simulink model "Lookuptabe1"  (R2025b)
settings: Solver=FixedStepDiscrete  StartTime=0.0  StopTime=1  FixedStep=0.0001  RelTol=1e-3
values from neighbouring files (symbols this model uses):
  A = 0.6*Xg.^2 - 0.4*Yg + 1.8*sin(2*Zg) + 0.15*Xg.*Yg.*sin(Zg) - 2.5    [test.m]    (also in test2.m = reshape(1:64, [4, 4, 4]))
  A1 = A(:)    [test.m]    (also in test2.m)
  X_dim = length(X_index)    [test.m]    (also in test2.m)
  X_index = linspace(-8.5, 12.3, 25)    [test.m]    (also in test2.m = X_index - 1.2)
  X_min = min(X_index)    [test.m]    (also in test2.m)
  X_step = X_index(2) - X_index(1)    [test.m]    (also in test2.m)
  XY_dim = X_dim * Y_dim    [test.m]    (also in test2.m)
  Y_dim = length(Y_index)    [test.m]    (also in test2.m)
  Y_index = linspace(-45.7, 67.2, 25)    [test.m]    (also in test2.m = Y_index - 2)
  Y_min = min(Y_index)    [test.m]    (also in test2.m)
  Y_step = Y_index(2) - Y_index(1)    [test.m]    (also in test2.m)
  Z_dim = length(Z_index)    [test.m]    (also in test2.m)
  Z_index = linspace(-3.8, 4.1, 25)    [test.m]    (also in test2.m = Z_index - 1)
  Z_min = min(Z_index)    [test.m]    (also in test2.m)
  Z_step = Z_index(2) - Z_index(1)    [test.m]    (also in test2.m)
settings Model: Creator=LXL1231A  LastModifiedBy=LXL1231A
settings OptimizationCC: DefaultParameterBehavior=Inlined  EnhancedBackFolding=on  PassReuseOutputArgsAs=Individual arguments  ZeroExternalMemoryAtStartup=off  ZeroInternalMemoryAtStartup=off  OptimizeBlockOrder=speed  DifferentSizesBufferReuse=on  OptimizationCustomize=off  EfficientTunableParamExpr=on
settings DebuggingCC: ParameterTunabilityLossMsg=error
settings SFSimCC: MATLABDynamicMemAlloc=off
settings RTWCC: SystemTargetFile=ert.tlc  GenCodeOnly=on  TemplateMakefile=ert_default_tmf  Description=Embedded Coder
settings CodeAppCC: ForceParamTrailComments=on  IgnoreCustomStorageClasses=off  OperatorAnnotations=on  SimulinkDataObjDesc=on  SFDataObjDesc=on  InsertBlockDesc=on
settings ERTTargetCC: ERTCustomFileTemplate=example_file_process.tlc  TargetLangStandard=C99 (ISO)  GenerateSampleERTMain=on

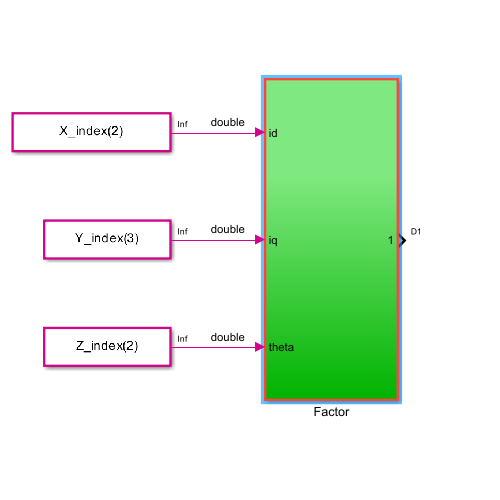
[thumbnail: Simulink's stored preview of the top-level diagram]
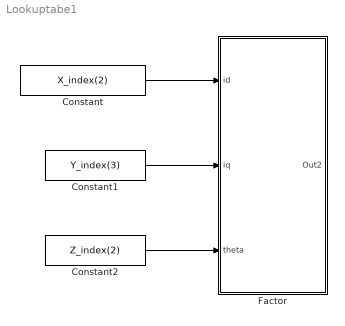
== system Lookuptabe1 ==
  Constant : Constant  Value=X_index(2)
  Constant1 : Constant  Value=Y_index(3)
  Constant2 : Constant  Value=Z_index(2)
  Factor : Subsystem
  wires:
  Constant/1 -> Factor/1(id)
  Constant1/1 -> Factor/2(iq)
  Constant2/1 -> Factor/3(theta)

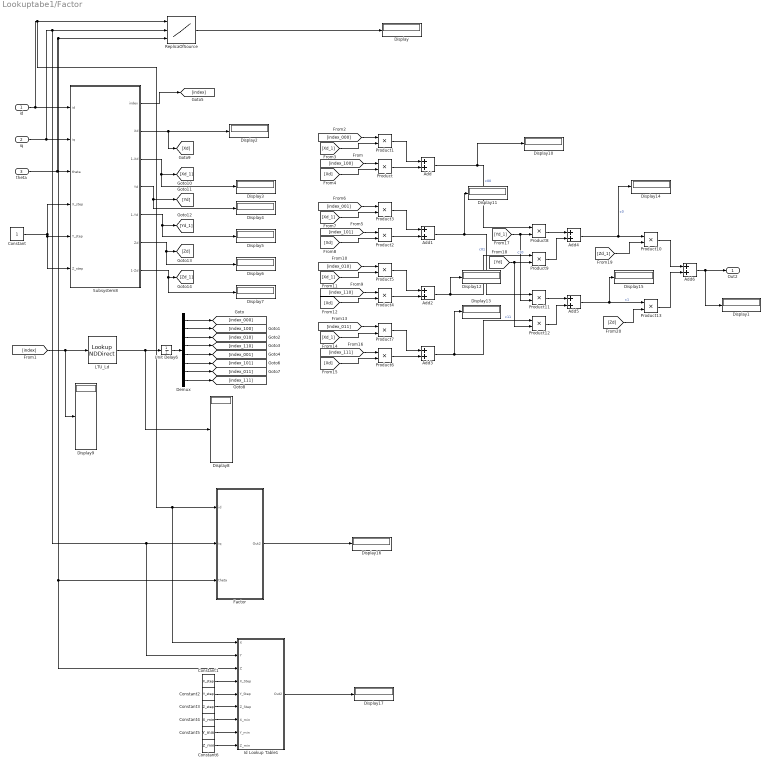
== system Lookuptabe1/Factor ==
  id : Inport
  iq : Inport  Port=2
  theta : Inport  Port=3
  Add{,1..6} (7 alike) : Sum
  Constant : Constant
  Constant1 : Constant  Value=X_step
  Constant2 : Constant  Value=Y_step
  Constant3 : Constant  Value=Z_step
  Constant4 : Constant  Value=X_min
  Constant5 : Constant  Value=Y_min
  Constant6 : Constant  Value=Z_min
  Demux : Demux  Outputs=8
  Display{,1..17} (18 alike) : Display
  Factor : Subsystem
  Id Lookup Table1 : Subsystem
  LTU_Ld : LookupNDDirect  NumberOfTableDimensions=1  Table=A1  TableDataTypeStr=fixdt(0,16,8)
  Product{,1..13} (14 alike) : Product
  ReplicaOfSource : Lookup_n-D  NumberOfTableDimensions=3  BreakpointsForDimension1=X_index  BreakpointsForDimension2=Y_index  BreakpointsForDimension3=Z_index  Table=A  InterpMethod=Linear Lagrange  InternalRulePriority=Speed  RndMeth=Simplest
      settings: InputPortMap=u0,u1,u2
  Subsystem8 : Subsystem
  Unit Delay6 : UnitDelay  SampleTime=-1  HasFrameUpgradeWarning=on
  Out2 : Outport
  wires:
  [index] -> Display9/1, LTU_Ld/1
  Subsystem8/1(index) -> [index]
  ReplicaOfSource/1 -> Display/1
  Constant/1 -> Subsystem8/6(Z_step), Subsystem8/5(Y_step), Subsystem8/4(X_step)
  Unit Delay6/1 -> Demux/1
  Demux/1 -> [index_000]
  [index_100] -> Product/1
  Product/1 -> Add/2
  Product1/1 -> Add/1
  [index_000] -> Product1/1
  Demux/2 -> [index_100]
  Demux/3 -> [index_010]
  Demux/4 -> [index_110]
  Demux/5 -> [index_001]
  Demux/6 -> [index_101]
  Demux/7 -> [index_011]
  Demux/8 -> [index_111]
  Subsystem8/2(Xd) -> [Xd], Display2/1
  Subsystem8/3(1-Xd) -> Display3/1, [Xd_1]
  Subsystem8/4(Yd) -> Display4/1, [Yd]
  Subsystem8/5(1-Yd) -> Display5/1, [Yd_1]
  Subsystem8/6(Zd) -> Display6/1, [Zd]
  Subsystem8/7(1-Zd) -> Display7/1, [Zd_1]
  [Xd_1] -> Product1/2
  [Xd] -> Product/2
  [index_101] -> Product2/1
  Product3/1 -> Add1/1
  Product2/1 -> Add1/2
  [index_001] -> Product3/1
  [Xd] -> Product2/2
  [Xd_1] -> Product3/2
  [index_010] -> Product5/1
  Product4/1 -> Add2/2
  Product5/1 -> Add2/1
  [Xd] -> Product4/2
  [index_110] -> Product4/1
  [Xd_1] -> Product5/2
  [Xd] -> Product6/2
  [index_111] -> Product6/1
  [index_011] -> Product7/1
  Product7/1 -> Add3/1
  Product6/1 -> Add3/2
  [Xd_1] -> Product7/2
  Add/1 -> Display10/1, Product8/1  "c00"
  [Yd_1] -> Product11/2, Product8/2
  Product8/1 -> Add4/1
  Product9/1 -> Add4/2
  Add2/1 -> Display12/1, Product9/1  "c10"
  [Yd] -> Product12/2, Product9/2
  Add4/1 -> Display14/1, Product10/1  "c0"
  [Zd_1] -> Product10/2
  Add1/1 -> Display11/1, Product11/1  "c01"
  Product11/1 -> Add5/1
  Add3/1 -> Display13/1, Product12/1  "c11"
  Product12/1 -> Add5/2
  Add5/1 -> Display15/1, Product13/1  "c1"
  [Zd] -> Product13/2
  Product10/1 -> Add6/1
  Product13/1 -> Add6/2
  Add6/1 -> Display1/1, Out2/1
  LTU_Ld/1 -> Display8/1, Unit Delay6/1
  Factor/1(Out2) -> Display16/1
  Constant1/1 -> Id Lookup Table1/4(X_Step)
  Id Lookup Table1/1(Out2) -> Display17/1
  Constant2/1 -> Id Lookup Table1/5(Y_Step)
  Constant3/1 -> Id Lookup Table1/6(Z_Step)
  Constant4/1 -> Id Lookup Table1/7(X_min)
  Constant5/1 -> Id Lookup Table1/8(Y_min)
  Constant6/1 -> Id Lookup Table1/9(Z_min)
  id/1 -> ReplicaOfSource/1, Id Lookup Table1/1(X), Factor/1(id), Subsystem8/1(id)
  iq/1 -> ReplicaOfSource/2, Id Lookup Table1/2(Y), Factor/2(iq), Subsystem8/2(iq)
  theta/1 -> ReplicaOfSource/3, Id Lookup Table1/3(Z), Factor/3(theta), Subsystem8/3(theta)

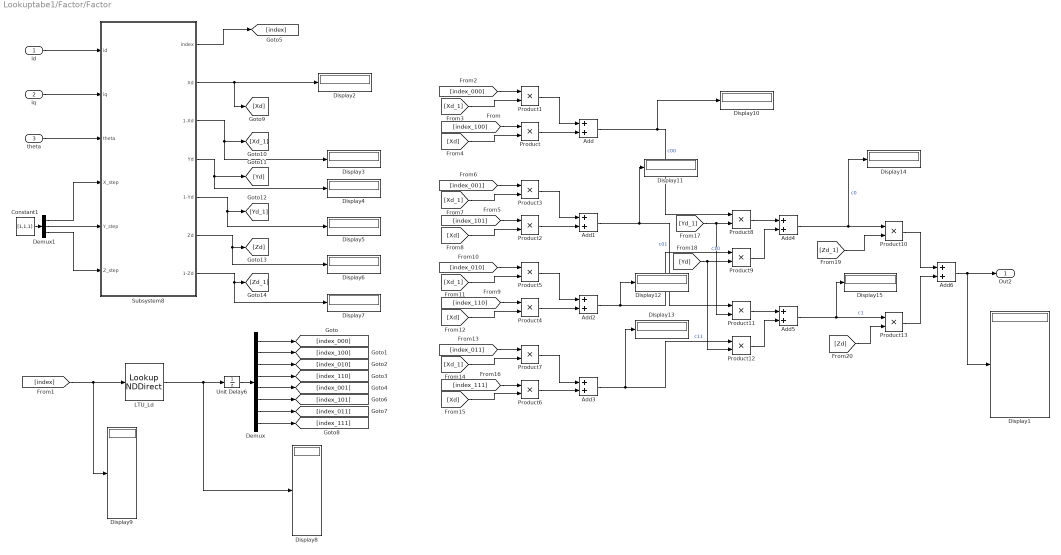
== system Lookuptabe1/Factor/Factor ==
  id : Inport
  iq : Inport  Port=2
  theta : Inport  Port=3
  Add{,1..6} (7 alike) : Sum
  Constant1 : Constant  Value=[1,1,1]
  Demux : Demux  Outputs=8
  Demux1 : Demux  Outputs=3
  Display{1..15} (15 alike) : Display
  LTU_Ld : LookupNDDirect  NumberOfTableDimensions=1  Table=A1  TableDataTypeStr=single
  Product{,1..13} (14 alike) : Product
  Subsystem8 : Subsystem
  Unit Delay6 : UnitDelay  SampleTime=-1  HasFrameUpgradeWarning=on
  Out2 : Outport
  wires:
  LTU_Ld/1 -> Unit Delay6/1, Display8/1
  Add6/1 -> Out2/1, Display1/1
  Product13/1 -> Add6/2
  Product10/1 -> Add6/1
  [Zd] -> Product13/2
  Add5/1 -> Product13/1, Display15/1  "c1"
  Product12/1 -> Add5/2
  Add3/1 -> Product12/1, Display13/1  "c11"
  Product11/1 -> Add5/1
  Add1/1 -> Product11/1, Display11/1  "c01"
  [Zd_1] -> Product10/2
  Add4/1 -> Product10/1, Display14/1  "c0"
  [Yd] -> Product9/2, Product12/2
  Add2/1 -> Product9/1, Display12/1  "c10"
  Product9/1 -> Add4/2
  Product8/1 -> Add4/1
  [Yd_1] -> Product8/2, Product11/2
  Add/1 -> Product8/1, Display10/1  "c00"
  [Xd_1] -> Product7/2
  Product6/1 -> Add3/2
  Product7/1 -> Add3/1
  [index_011] -> Product7/1
  [index_111] -> Product6/1
  [Xd] -> Product6/2
  [Xd_1] -> Product5/2
  [index_110] -> Product4/1
  [Xd] -> Product4/2
  Product5/1 -> Add2/1
  Product4/1 -> Add2/2
  [index_010] -> Product5/1
  [Xd_1] -> Product3/2
  [Xd] -> Product2/2
  [index_001] -> Product3/1
  Product2/1 -> Add1/2
  Product3/1 -> Add1/1
  [index_101] -> Product2/1
  [Xd] -> Product/2
  [Xd_1] -> Product1/2
  Subsystem8/7(1-Zd) -> [Zd_1], Display7/1
  Subsystem8/6(Zd) -> [Zd], Display6/1
  Subsystem8/5(1-Yd) -> [Yd_1], Display5/1
  Subsystem8/4(Yd) -> [Yd], Display4/1
  Subsystem8/3(1-Xd) -> [Xd_1], Display3/1
  Subsystem8/2(Xd) -> Display2/1, [Xd]
  Demux/8 -> [index_111]
  Demux/7 -> [index_011]
  Demux/6 -> [index_101]
  Demux/5 -> [index_001]
  Demux/4 -> [index_110]
  Demux/3 -> [index_010]
  Demux/2 -> [index_100]
  [index_000] -> Product1/1
  Product1/1 -> Add/1
  Product/1 -> Add/2
  [index_100] -> Product/1
  Demux/1 -> [index_000]
  Unit Delay6/1 -> Demux/1
  Subsystem8/1(index) -> [index]
  theta/1 -> Subsystem8/3(theta)
  iq/1 -> Subsystem8/2(iq)
  id/1 -> Subsystem8/1(id)
  [index] -> LTU_Ld/1, Display9/1
  Constant1/1 -> Demux1/1
  Demux1/1 -> Subsystem8/4(X_step)
  Demux1/2 -> Subsystem8/5(Y_step)
  Demux1/3 -> Subsystem8/6(Z_step)

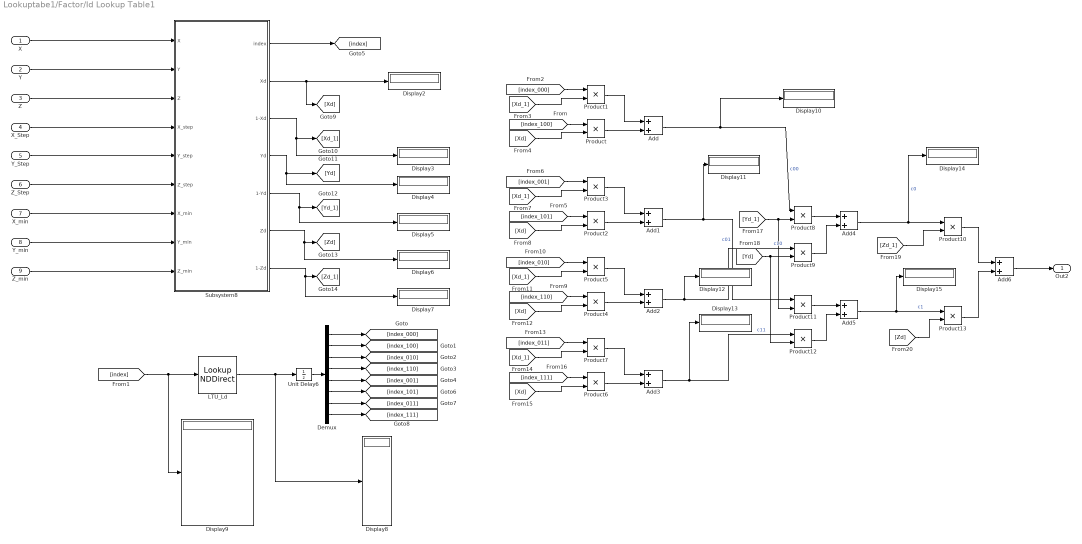
== system Lookuptabe1/Factor/Id Lookup Table1 ==
  X : Inport
  Y : Inport  Port=2
  Z : Inport  Port=3
  X_Step : Inport  Port=4
  Y_Step : Inport  Port=5
  Z_Step : Inport  Port=6
  X_min : Inport  Port=7
  Y_min : Inport  Port=8
  Z_min : Inport  Port=9
  Add{,1..6} (7 alike) : Sum
  Demux : Demux  Outputs=8
  Display{2..15} (14 alike) : Display
  LTU_Ld : LookupNDDirect  NumberOfTableDimensions=1  Table=A1  TableDataTypeStr=single
  Product{,1..13} (14 alike) : Product
  Subsystem8 : Subsystem
  Unit Delay6 : UnitDelay  SampleTime=-1  HasFrameUpgradeWarning=on
  Out2 : Outport
  wires:
  [index] -> Display9/1, LTU_Ld/1
  X/1 -> Subsystem8/1(X)
  Y/1 -> Subsystem8/2(Y)
  Z/1 -> Subsystem8/3(Z)
  Subsystem8/1(index) -> [index]
  Unit Delay6/1 -> Demux/1
  Demux/1 -> [index_000]
  [index_100] -> Product/1
  Product/1 -> Add/2
  Product1/1 -> Add/1
  [index_000] -> Product1/1
  Demux/2 -> [index_100]
  Demux/3 -> [index_010]
  Demux/4 -> [index_110]
  Demux/5 -> [index_001]
  Demux/6 -> [index_101]
  Demux/7 -> [index_011]
  Demux/8 -> [index_111]
  Subsystem8/2(Xd) -> [Xd], Display2/1
  Subsystem8/3(1-Xd) -> Display3/1, [Xd_1]
  Subsystem8/4(Yd) -> Display4/1, [Yd]
  Subsystem8/5(1-Yd) -> Display5/1, [Yd_1]
  Subsystem8/6(Zd) -> Display6/1, [Zd]
  Subsystem8/7(1-Zd) -> Display7/1, [Zd_1]
  [Xd_1] -> Product1/2
  [Xd] -> Product/2
  [index_101] -> Product2/1
  Product3/1 -> Add1/1
  Product2/1 -> Add1/2
  [index_001] -> Product3/1
  [Xd] -> Product2/2
  [Xd_1] -> Product3/2
  [index_010] -> Product5/1
  Product4/1 -> Add2/2
  Product5/1 -> Add2/1
  [Xd] -> Product4/2
  [index_110] -> Product4/1
  [Xd_1] -> Product5/2
  [Xd] -> Product6/2
  [index_111] -> Product6/1
  [index_011] -> Product7/1
  Product7/1 -> Add3/1
  Product6/1 -> Add3/2
  [Xd_1] -> Product7/2
  Add/1 -> Display10/1, Product8/1  "c00"
  [Yd_1] -> Product11/2, Product8/2
  Product8/1 -> Add4/1
  Product9/1 -> Add4/2
  Add2/1 -> Display12/1, Product9/1  "c10"
  [Yd] -> Product12/2, Product9/2
  Add4/1 -> Display14/1, Product10/1  "c0"
  [Zd_1] -> Product10/2
  Add1/1 -> Display11/1, Product11/1  "c01"
  Product11/1 -> Add5/1
  Add3/1 -> Display13/1, Product12/1  "c11"
  Product12/1 -> Add5/2
  Add5/1 -> Display15/1, Product13/1  "c1"
  [Zd] -> Product13/2
  Product10/1 -> Add6/1
  Product13/1 -> Add6/2
  Add6/1 -> Out2/1
  LTU_Ld/1 -> Display8/1, Unit Delay6/1
  X_Step/1 -> Subsystem8/4(X_step)
  Y_Step/1 -> Subsystem8/5(Y_step)
  Z_Step/1 -> Subsystem8/6(Z_step)
  X_min/1 -> Subsystem8/7(X_min)
  Z_min/1 -> Subsystem8/9(Z_min)
  Y_min/1 -> Subsystem8/8(Y_min)

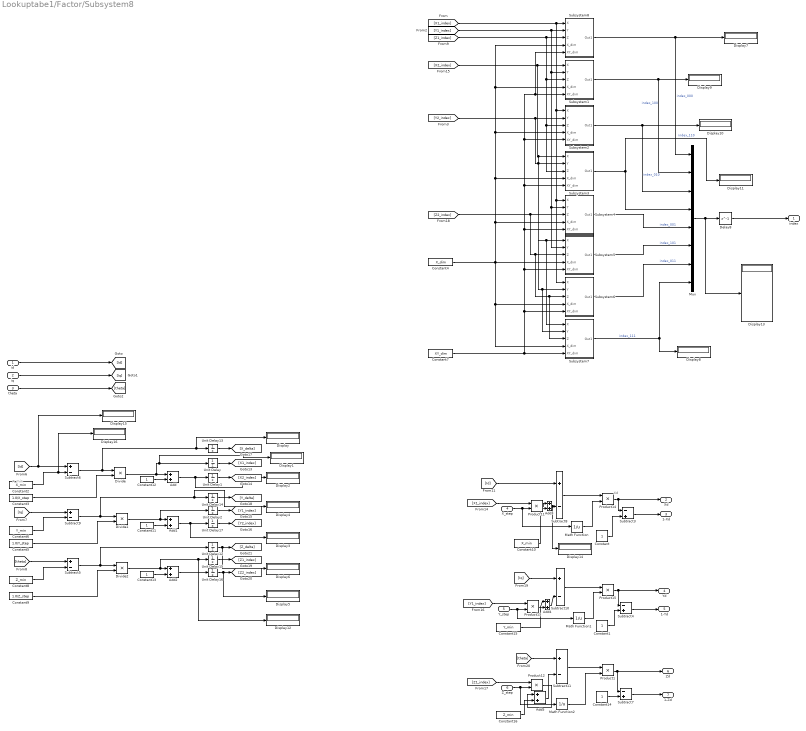
== system Lookuptabe1/Factor/Subsystem8 ==
  note: Xd
  note: X_min
  id : Inport
  iq : Inport  Port=2
  theta : Inport  Port=3
  X_step : Inport  Port=4
  Y_step : Inport  Port=5
  Z_step : Inport  Port=6
  Add : Sum  OutDataTypeStr=uint16
  Add1 : Sum  OutDataTypeStr=uint16
  Add2 : Sum  OutDataTypeStr=uint16
  Add3 : Sum
  Add4 : Sum
  Add5 : Sum
  Constant : Constant
  Constant1 : Constant
  Constant10 : Constant  Value=X_min  OutDataTypeStr=fixdt(1,LdLqTable_len,LdLqTable_fac)  SampleTime=-1
  Constant11 : Constant  OutDataTypeStr=uint16  SampleTime=-1
  Constant12 : Constant  OutDataTypeStr=uint16  SampleTime=-1
  Constant13 : Constant  OutDataTypeStr=uint16  SampleTime=-1
  Constant14 : Constant
  Constant15 : Constant  Value=Y_min  OutDataTypeStr=fixdt(1,LdLqTable_len,LdLqTable_fac)  SampleTime=-1
  Constant16 : Constant  Value=Z_min  OutDataTypeStr=fixdt(1,LdLqTable_len,LdLqTable_fac)  SampleTime=-1
  Constant2 : Constant  Value=X_min  OutDataTypeStr=fixdt(1,LdLqTable_len,LdLqTable_fac)  SampleTime=-1
  Constant3 : Constant  Value=1.0/X_step  OutDataTypeStr=fixdt(1,LdLqTable_len,LdLqTable_fac)  SampleTime=-1
  Constant4 : Constant  Value=X_dim  OutDataTypeStr=uint16  SampleTime=-1
  Constant5 : Constant  Value=1.0/Y_step  OutDataTypeStr=fixdt(1,LdLqTable_len,LdLqTable_fac)  SampleTime=-1
  Constant6 : Constant  Value=Y_min  OutDataTypeStr=fixdt(1,LdLqTable_len,LdLqTable_fac)  SampleTime=-1
  Constant7 : Constant  Value=XY_dim  OutDataTypeStr=uint16  SampleTime=-1
  Constant8 : Constant  Value=Z_min  OutDataTypeStr=fixdt(1,LdLqTable_len,LdLqTable_fac)  SampleTime=-1
  Constant9 : Constant  Value=1.0/Z_step  OutDataTypeStr=fixdt(1,LdLqTable_len,LdLqTable_fac)  SampleTime=-1
  Delay8 : Delay  DelayLength=1
  Display{,1..16} (17 alike) : Display
  Divide : Product  OutDataTypeStr=uint16
  Divide1 : Product  OutDataTypeStr=uint16
  Divide2 : Product  OutDataTypeStr=uint16
  Math Function : Math  Operator=reciprocal
  Math Function1 : Math  Operator=reciprocal
  Math Function2 : Math  Operator=reciprocal
  Mux : Mux  Inputs=8
  Product1 : Product
  Product11 : Product  OutDataTypeStr=fixdt(1,LdLqTable_len,LdLqTable_fac)
  Product12 : Product  OutDataTypeStr=fixdt(1,LdLqTable_len,LdLqTable_fac)
  Product13 : Product  OutDataTypeStr=fixdt(1,LdLqTable_len,LdLqTable_fac)
  Product14 : Product
  Product15 : Product
  Subsystem1 : Subsystem
  Subsystem2 : Subsystem
  Subsystem3 : Subsystem
  Subsystem4 : Subsystem
  Subsystem5 : Subsystem
  Subsystem6 : Subsystem
  Subsystem7 : Subsystem
  Subsystem8 : Subsystem
  Subtract10 : Sum  Inputs=+-  OutDataTypeStr=fixdt(1,LdLqTable_len,LdLqTable_fac)
  Subtract11 : Sum  Inputs=+-  OutDataTypeStr=fixdt(1,LdLqTable_len,LdLqTable_fac)
  Subtract3 : Sum  Inputs=-+
  Subtract4 : Sum  Inputs=-+
  Subtract5 : Sum  Inputs=+-  OutDataTypeStr=fixdt(1,Id_lim_len,Id_lim_fac)
  Subtract6 : Sum  Inputs=+-  OutDataTypeStr=fixdt(1,Id_lim_len,Id_lim_fac)
  Subtract7 : Sum  Inputs=-+
  Subtract8 : Sum  Inputs=+-  OutDataTypeStr=fixdt(1,LdLqTable_len,LdLqTable_fac)
  Subtract9 : Sum  Inputs=+-  OutDataTypeStr=fixdt(1,Id_lim_len,Id_lim_fac)
  Unit Delay{,1..2,12..17} (9 alike) : UnitDelay  SampleTime=-1  HasFrameUpgradeWarning=on
  index : Outport
  Xd : Outport  Port=2
  1-Xd : Outport  Port=3
  Yd : Outport  Port=4
  1-Yd : Outport  Port=5
  Zd : Outport  Port=6
  1-Zd : Outport  Port=7
  wires:
  Constant9/1 -> Divide2/2
  Subtract6/1 -> Display/1, Unit Delay13/1, Divide/1
  Mux/1 -> Display13/1, Delay8/1
  Unit Delay16/1 -> Display5/1, [Z2_index]
  [Z2_index] -> Subsystem4/3(Z), Subsystem5/3(Z), Subsystem7/3(Z), Subsystem6/3(Z)
  [X1_index] -> Subsystem8/1(X), Subsystem2/1(X), Subsystem6/1(X), Subsystem4/1(X)
  Divide/1 -> Unit Delay/1, Display1/1, Add/1
  Constant8/1 -> Subtract5/2
  Unit Delay2/1 -> [Y1_index]
  Unit Delay13/1 -> [X_delta]
  Constant4/1 -> Subsystem8/4(X_dim), Subsystem1/4(X_dim), Subsystem2/4(X_dim), Subsystem3/4(X_dim), Subsystem4/4(X_dim), Subsystem5/4(X_dim), Subsystem7/4(X_dim), Subsystem6/4(X_dim)
  Unit Delay12/1 -> Display6/1, [Z_delta]
  Constant7/1 -> Subsystem6/5(XY_dim), Subsystem5/5(XY_dim), Subsystem4/5(XY_dim), Subsystem3/5(XY_dim), Subsystem2/5(XY_dim), Subsystem1/5(XY_dim), Subsystem8/5(XY_dim), Subsystem7/5(XY_dim)
  Constant13/1 -> Add2/2
  Divide1/1 -> Unit Delay2/1, Add1/1
  Constant12/1 -> Add/2
  [Y2_index] -> Subsystem2/2(Y), Subsystem3/2(Y), Subsystem7/2(Y), Subsystem6/2(Y)
  Subtract9/1 -> Divide1/1, Display4/1, Unit Delay14/1
  Unit Delay/1 -> [X1_index]
  Constant11/1 -> Add1/2
  Unit Delay1/1 -> [X2_index]
  Unit Delay15/1 -> [Z1_index]
  Subsystem2/1(Out1) -> Display10/1, Mux/3  "index_010"
  Subsystem8/1(Out1) -> Display7/1, Mux/1  "index_000"
  Add1/1 -> Display3/1, Unit Delay17/1
  Constant2/1 -> Display16/1, Subtract6/2
  Subsystem1/1(Out1) -> Display9/1, Mux/2  "index_100"
  Unit Delay14/1 -> [Y_delta]
  Subsystem3/1(Out1) -> Mux/4, Display11/1  "index_110"
  [X2_index] -> Subsystem1/1(X), Subsystem3/1(X), Subsystem7/1(X), Subsystem5/1(X)
  Constant6/1 -> Subtract9/2
  Unit Delay17/1 -> [Y2_index]
  Constant3/1 -> Divide/2
  Subsystem7/1(Out1) -> Mux/8, Display8/1  "index_111"
  [Z1_index] -> Subsystem8/3(Z), Subsystem1/3(Z), Subsystem3/3(Z), Subsystem2/3(Z)
  Constant5/1 -> Divide1/2
  Add/1 -> Display2/1, Unit Delay1/1
  Delay8/1 -> index/1
  Subtract5/1 -> Divide2/1, Unit Delay12/1
  Add2/1 -> Unit Delay16/1
  Subsystem6/1(Out1) -> Mux/7  "index_011"
  Subsystem4/1(Out1) -> Mux/5  "index_001"
  [Y1_index] -> Subsystem8/2(Y), Subsystem1/2(Y), Subsystem5/2(Y), Subsystem4/2(Y)
  Divide2/1 -> Display12/1, Unit Delay15/1, Add2/1
  Subsystem5/1(Out1) -> Mux/6  "index_101"
  [Iq] -> Subtract9/1
  [theta] -> Subtract5/1
  id/1 -> [Id]
  iq/1 -> [Iq]
  theta/1 -> [theta]
  [Id] -> Subtract8/1
  Product11/1 -> Add3/1
  [theta] -> Subtract11/1
  [X1_index] -> Product11/1
  Y_step/1 -> Math Function1/1, Product13/2
  [Iq] -> Subtract10/1
  Z_step/1 -> Math Function2/1, Product12/2
  Product12/1 -> Add5/1
  X_step/1 -> Math Function/1, Product11/2
  [Y1_index] -> Product13/1
  [Z1_index] -> Product12/1
  Product13/1 -> Add4/1
  Subtract8/1 -> Product14/1
  Math Function/1 -> Product14/2
  Subtract10/1 -> Product15/1
  Math Function1/1 -> Product15/2
  Math Function2/1 -> Product1/2
  Subtract11/1 -> Product1/1
  Product14/1 -> Subtract3/1, Xd/1
  Product15/1 -> Subtract4/1, Yd/1
  Product1/1 -> Subtract7/1, Zd/1
  Subtract3/1 -> 1-Xd/1
  Constant/1 -> Subtract3/2
  Subtract4/1 -> 1-Yd/1
  Constant1/1 -> Subtract4/2
  Subtract7/1 -> 1-Zd/1
  Constant14/1 -> Subtract7/2
  Add3/1 -> Display14/1, Subtract8/2
  Constant10/1 -> Add3/2
  Add4/1 -> Subtract10/2
  Constant15/1 -> Add4/2
  Constant16/1 -> Add5/2
  Add5/1 -> Subtract11/2
  [Id] -> Display15/1, Subtract6/1

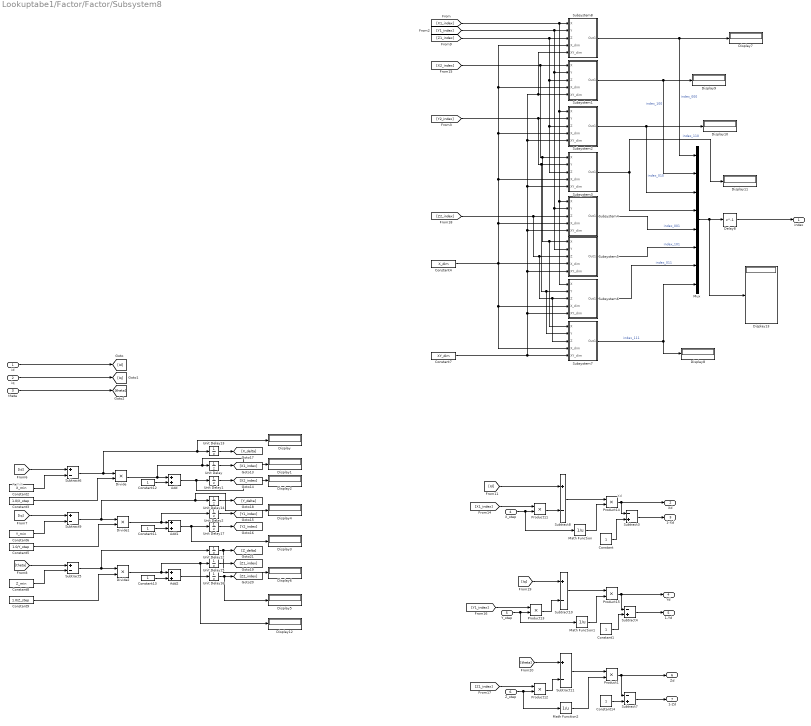
== system Lookuptabe1/Factor/Factor/Subsystem8 ==
  note: X_min
  note: Xd
  id : Inport
  iq : Inport  Port=2
  theta : Inport  Port=3
  X_step : Inport  Port=4
  Y_step : Inport  Port=5
  Z_step : Inport  Port=6
  Add : Sum
  Add1 : Sum  OutDataTypeStr=single
  Add2 : Sum  OutDataTypeStr=single  AccumDataTypeStr=single
  Constant : Constant
  Constant1 : Constant
  Constant11 : Constant  OutDataTypeStr=uint32  SampleTime=-1
  Constant12 : Constant  OutDataTypeStr=uint32  SampleTime=-1
  Constant13 : Constant  OutDataTypeStr=uint32  SampleTime=-1
  Constant14 : Constant
  Constant2 : Constant  Value=X_min  OutDataTypeStr=single  SampleTime=-1
  Constant3 : Constant  Value=1.0/X_step  OutDataTypeStr=single  SampleTime=-1
  Constant4 : Constant  Value=X_dim  OutDataTypeStr=single  SampleTime=-1
  Constant5 : Constant  Value=1.0/Y_step  OutDataTypeStr=single  SampleTime=-1
  Constant6 : Constant  Value=Y_min  OutDataTypeStr=single  SampleTime=-1
  Constant7 : Constant  Value=XY_dim  OutDataTypeStr=single  SampleTime=-1
  Constant8 : Constant  Value=Z_min  OutDataTypeStr=single  SampleTime=-1
  Constant9 : Constant  Value=1.0/Z_step  OutDataTypeStr=single  SampleTime=-1
  Delay8 : Delay  DelayLength=1
  Display{,1..13} (14 alike) : Display
  Divide : Product  OutDataTypeStr=uint16
  Divide1 : Product  OutDataTypeStr=uint16
  Divide2 : Product  OutDataTypeStr=uint16
  Math Function : Math  Operator=reciprocal
  Math Function1 : Math  Operator=reciprocal
  Math Function2 : Math  Operator=reciprocal
  Mux : Mux  Inputs=8
  Product1 : Product
  Product11 : Product  OutDataTypeStr=single
  Product12 : Product  OutDataTypeStr=single
  Product13 : Product  OutDataTypeStr=single
  Product14 : Product
  Product15 : Product
  Subsystem1 : Subsystem
  Subsystem2 : Subsystem
  Subsystem3 : Subsystem
  Subsystem4 : Subsystem
  Subsystem5 : Subsystem
  Subsystem6 : Subsystem
  Subsystem7 : Subsystem
  Subsystem8 : Subsystem
  Subtract{5..6,8..11} (6 alike) : Sum  Inputs=+-  OutDataTypeStr=single
  Subtract3 : Sum  Inputs=-+
  Subtract4 : Sum  Inputs=-+
  Subtract7 : Sum  Inputs=-+
  Unit Delay{,1..2,12..17} (9 alike) : UnitDelay  SampleTime=-1  HasFrameUpgradeWarning=on
  index : Outport
  Xd : Outport  Port=2
  1-Xd : Outport  Port=3
  Yd : Outport  Port=4
  1-Yd : Outport  Port=5
  Zd : Outport  Port=6
  1-Zd : Outport  Port=7
  wires:
  Constant14/1 -> Subtract7/2
  Subtract7/1 -> 1-Zd/1
  Constant1/1 -> Subtract4/2
  Subtract4/1 -> 1-Yd/1
  Constant/1 -> Subtract3/2
  Subtract3/1 -> 1-Xd/1
  Product1/1 -> Zd/1, Subtract7/1
  Product15/1 -> Yd/1, Subtract4/1
  Product14/1 -> Xd/1, Subtract3/1
  Subtract11/1 -> Product1/1
  Math Function2/1 -> Product1/2
  Math Function1/1 -> Product15/2
  Subtract10/1 -> Product15/1
  Math Function/1 -> Product14/2
  Subtract8/1 -> Product14/1
  Product13/1 -> Subtract10/2
  [Z1_index] -> Product12/1
  [Y1_index] -> Product13/1
  X_step/1 -> Product11/2, Math Function/1
  Product12/1 -> Subtract11/2
  Z_step/1 -> Product12/2, Math Function2/1
  [Iq] -> Subtract10/1
  Y_step/1 -> Product13/2, Math Function1/1
  [X1_index] -> Product11/1
  [theta] -> Subtract11/1
  Product11/1 -> Subtract8/2
  [Id] -> Subtract8/1
  theta/1 -> [theta]
  iq/1 -> [Iq]
  id/1 -> [Id]
  [theta] -> Subtract5/1
  [Iq] -> Subtract9/1
  [Id] -> Subtract6/1
  Subsystem5/1(Out1) -> Mux/6  "index_101"
  Divide2/1 -> Add2/1, Unit Delay15/1, Display12/1
  [Y1_index] -> Subsystem5/2(Y), Subsystem4/2(Y), Subsystem1/2(Y), Subsystem8/2(Y)
  Subsystem4/1(Out1) -> Mux/5  "index_001"
  Subsystem6/1(Out1) -> Mux/7  "index_011"
  Add2/1 -> Unit Delay16/1
  Subtract5/1 -> Unit Delay12/1, Divide2/1
  Delay8/1 -> index/1
  Add/1 -> Unit Delay1/1, Display2/1
  Constant5/1 -> Divide1/2
  [Z1_index] -> Subsystem3/3(Z), Subsystem2/3(Z), Subsystem1/3(Z), Subsystem8/3(Z)
  Subsystem7/1(Out1) -> Display8/1, Mux/8  "index_111"
  Constant3/1 -> Divide/2
  Unit Delay17/1 -> [Y2_index]
  Constant6/1 -> Subtract9/2
  [X2_index] -> Subsystem3/1(X), Subsystem7/1(X), Subsystem5/1(X), Subsystem1/1(X)
  Subsystem3/1(Out1) -> Display11/1, Mux/4  "index_110"
  Unit Delay14/1 -> [Y_delta]
  Subsystem1/1(Out1) -> Mux/2, Display9/1  "index_100"
  Constant2/1 -> Subtract6/2
  Add1/1 -> Unit Delay17/1, Display3/1
  Subsystem8/1(Out1) -> Mux/1, Display7/1  "index_000"
  Subsystem2/1(Out1) -> Mux/3, Display10/1  "index_010"
  Unit Delay15/1 -> [Z1_index]
  Unit Delay1/1 -> [X2_index]
  Constant11/1 -> Add1/2
  Unit Delay/1 -> [X1_index]
  Subtract9/1 -> Unit Delay14/1, Display4/1, Divide1/1
  [Y2_index] -> Subsystem2/2(Y), Subsystem3/2(Y), Subsystem7/2(Y), Subsystem6/2(Y)
  Constant12/1 -> Add/2
  Divide1/1 -> Add1/1, Unit Delay2/1
  Constant13/1 -> Add2/2
  Constant7/1 -> Subsystem7/5(XY_dim), Subsystem6/5(XY_dim), Subsystem5/5(XY_dim), Subsystem4/5(XY_dim), Subsystem3/5(XY_dim), Subsystem2/5(XY_dim), Subsystem8/5(XY_dim), Subsystem1/5(XY_dim)
  Unit Delay12/1 -> [Z_delta], Display6/1
  Constant4/1 -> Subsystem5/4(X_dim), Subsystem7/4(X_dim), Subsystem6/4(X_dim), Subsystem4/4(X_dim), Subsystem3/4(X_dim), Subsystem2/4(X_dim), Subsystem1/4(X_dim), Subsystem8/4(X_dim)
  Unit Delay13/1 -> [X_delta]
  Unit Delay2/1 -> [Y1_index]
  Constant8/1 -> Subtract5/2
  Divide/1 -> Add/1, Unit Delay/1, Display1/1
  [X1_index] -> Subsystem2/1(X), Subsystem6/1(X), Subsystem4/1(X), Subsystem8/1(X)
  [Z2_index] -> Subsystem4/3(Z), Subsystem5/3(Z), Subsystem7/3(Z), Subsystem6/3(Z)
  Unit Delay16/1 -> [Z2_index], Display5/1
  Mux/1 -> Delay8/1, Display13/1
  Subtract6/1 -> Divide/1, Unit Delay13/1, Display/1
  Constant9/1 -> Divide2/2

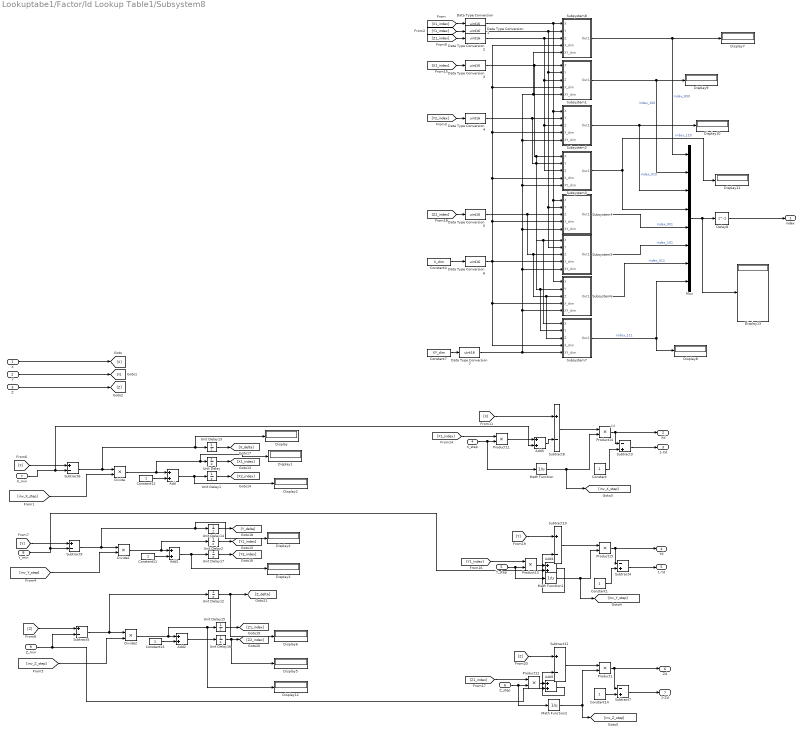
== system Lookuptabe1/Factor/Id Lookup Table1/Subsystem8 ==
  note: Xd
  X : Inport
  Y : Inport  Port=2
  Z : Inport  Port=3
  X_step : Inport  Port=4
  Y_step : Inport  Port=5
  Z_step : Inport  Port=6
  X_min : Inport  Port=7
  Y_min : Inport  Port=8
  Z_min : Inport  Port=9
  Add{,3..5} (4 alike) : Sum
  Add1 : Sum  OutDataTypeStr=single
  Add2 : Sum  OutDataTypeStr=single  AccumDataTypeStr=single
  Constant : Constant
  Constant1 : Constant
  Constant11 : Constant  OutDataTypeStr=uint32  SampleTime=-1
  Constant12 : Constant  OutDataTypeStr=uint32  SampleTime=-1
  Constant13 : Constant  OutDataTypeStr=uint32  SampleTime=-1
  Constant14 : Constant
  Constant4 : Constant  Value=X_dim  OutDataTypeStr=single  SampleTime=-1
  Constant7 : Constant  Value=XY_dim  OutDataTypeStr=single  SampleTime=-1
  Data Type Conversion{,1..7} (8 alike) : DataTypeConversion  OutDataTypeStr=uint16  SaturateOnIntegerOverflow=off  RndMeth=Floor
  Delay8 : Delay  DelayLength=1
  Display{,1..13} (14 alike) : Display
  Divide : Product  OutDataTypeStr=single
  Divide1 : Product  OutDataTypeStr=single
  Divide2 : Product  OutDataTypeStr=single
  Math Function : Math  Operator=reciprocal
  Math Function1 : Math  Operator=reciprocal
  Math Function2 : Math  Operator=reciprocal
  Mux : Mux  Inputs=8
  Product1 : Product
  Product11 : Product  OutDataTypeStr=single
  Product12 : Product  OutDataTypeStr=single
  Product13 : Product  OutDataTypeStr=single
  Product14 : Product
  Product15 : Product
  Subsystem1 : Subsystem
  Subsystem2 : Subsystem
  Subsystem3 : Subsystem
  Subsystem4 : Subsystem
  Subsystem5 : Subsystem
  Subsystem6 : Subsystem
  Subsystem7 : Subsystem
  Subsystem8 : Subsystem
  Subtract{5..6,8..11} (6 alike) : Sum  Inputs=+-  OutDataTypeStr=single
  Subtract3 : Sum  Inputs=-+
  Subtract4 : Sum  Inputs=-+
  Subtract7 : Sum  Inputs=-+
  Unit Delay{,1..2,12..17} (9 alike) : UnitDelay  SampleTime=-1  HasFrameUpgradeWarning=on
  index : Outport
  Xd : Outport  Port=2
  1-Xd : Outport  Port=3
  Yd : Outport  Port=4
  1-Yd : Outport  Port=5
  Zd : Outport  Port=6
  1-Zd : Outport  Port=7
  wires:
  [inv_Z_step] -> Divide2/2
  Subtract6/1 -> Display/1, Unit Delay13/1, Divide/1
  Mux/1 -> Display13/1, Delay8/1
  Unit Delay16/1 -> Display5/1, [Z2_index]
  [Z2_index] -> Data Type Conversion5/1
  [X1_index] -> Data Type Conversion/1
  Divide/1 -> Display1/1, Unit Delay/1, Add/1
  Unit Delay2/1 -> [Y1_index]
  Unit Delay13/1 -> [X_delta]
  Constant4/1 -> Data Type Conversion6/1
  Unit Delay12/1 -> Display6/1, [Z_delta]
  Constant7/1 -> Data Type Conversion7/1
  Constant13/1 -> Add2/2
  Divide1/1 -> Unit Delay2/1, Add1/1
  Constant12/1 -> Add/2
  [Y2_index] -> Data Type Conversion4/1
  Subtract9/1 -> Divide1/1, Display4/1, Unit Delay14/1
  Unit Delay/1 -> [X1_index]
  Constant11/1 -> Add1/2
  Unit Delay1/1 -> [X2_index]
  Unit Delay15/1 -> [Z1_index]
  Subsystem2/1(Out1) -> Display10/1, Mux/3  "index_010"
  Subsystem8/1(Out1) -> Display7/1, Mux/1  "index_000"
  Add1/1 -> Display3/1, Unit Delay17/1
  X_min/1 -> Add3/2, Subtract6/2
  Subsystem1/1(Out1) -> Display9/1, Mux/2  "index_100"
  Unit Delay14/1 -> [Y_delta]
  Subsystem3/1(Out1) -> Mux/4, Display11/1  "index_110"
  [X2_index] -> Data Type Conversion3/1
  Unit Delay17/1 -> [Y2_index]
  [inv_X_step] -> Divide/2
  Subsystem7/1(Out1) -> Mux/8, Display8/1  "index_111"
  [Z1_index] -> Data Type Conversion2/1
  [inv_Y_step] -> Divide1/2
  Add/1 -> Display2/1, Unit Delay1/1
  Delay8/1 -> index/1
  Subtract5/1 -> Divide2/1, Unit Delay12/1
  Add2/1 -> Unit Delay16/1
  Subsystem6/1(Out1) -> Mux/7  "index_011"
  Subsystem4/1(Out1) -> Mux/5  "index_001"
  [Y1_index] -> Data Type Conversion1/1
  Divide2/1 -> Display12/1, Unit Delay15/1, Add2/1
  Subsystem5/1(Out1) -> Mux/6  "index_101"
  [X] -> Subtract6/1
  [Y] -> Subtract9/1
  [Z] -> Subtract5/1
  X/1 -> [X]
  Y/1 -> [Y]
  Z/1 -> [Z]
  [X] -> Subtract8/1
  Product11/1 -> Add3/1
  [Z] -> Subtract11/1
  [X1_index] -> Product11/1
  Y_step/1 -> Math Function1/1, Product13/2
  [Y] -> Subtract10/1
  Z_step/1 -> Math Function2/1, Product12/2
  Product12/1 -> Add5/1
  X_step/1 -> Math Function/1, Product11/2
  [Y1_index] -> Product13/1
  [Z1_index] -> Product12/1
  Product13/1 -> Add4/1
  Subtract8/1 -> Product14/1
  Math Function/1 -> [inv_X_step], Product14/2
  Subtract10/1 -> Product15/1
  Math Function1/1 -> [inv_Y_step], Product15/2
  Math Function2/1 -> [inv_Z_step], Product1/2
  Subtract11/1 -> Product1/1
  Product14/1 -> Subtract3/1, Xd/1
  Product15/1 -> Subtract4/1, Yd/1
  Product1/1 -> Subtract7/1, Zd/1
  Subtract3/1 -> 1-Xd/1
  Constant/1 -> Subtract3/2
  Subtract4/1 -> 1-Yd/1
  Constant1/1 -> Subtract4/2
  Subtract7/1 -> 1-Zd/1
  Constant14/1 -> Subtract7/2
  Y_min/1 -> Add4/2, Subtract9/2
  Add3/1 -> Subtract8/2
  Add4/1 -> Subtract10/2
  Add5/1 -> Subtract11/2
  Z_min/1 -> Add5/2, Subtract5/2
  Data Type Conversion/1 -> Subsystem8/1(X), Subsystem4/1(X), Subsystem6/1(X), Subsystem2/1(X)
  Data Type Conversion1/1 -> Subsystem8/2(Y), Subsystem1/2(Y), Subsystem4/2(Y), Subsystem5/2(Y)
  Data Type Conversion2/1 -> Subsystem8/3(Z), Subsystem1/3(Z), Subsystem2/3(Z), Subsystem3/3(Z)
  Data Type Conversion3/1 -> Subsystem1/1(X), Subsystem5/1(X), Subsystem7/1(X), Subsystem3/1(X)
  Data Type Conversion4/1 -> Subsystem6/2(Y), Subsystem7/2(Y), Subsystem3/2(Y), Subsystem2/2(Y)
  Data Type Conversion5/1 -> Subsystem6/3(Z), Subsystem7/3(Z), Subsystem5/3(Z), Subsystem4/3(Z)
  Data Type Conversion6/1 -> Subsystem8/4(X_dim), Subsystem1/4(X_dim), Subsystem2/4(X_dim), Subsystem3/4(X_dim), Subsystem4/4(X_dim), Subsystem6/4(X_dim), Subsystem7/4(X_dim), Subsystem5/4(X_dim)
  Data Type Conversion7/1 -> Subsystem1/5(XY_dim), Subsystem8/5(XY_dim), Subsystem2/5(XY_dim), Subsystem3/5(XY_dim), Subsystem4/5(XY_dim), Subsystem5/5(XY_dim), Subsystem6/5(XY_dim), Subsystem7/5(XY_dim)

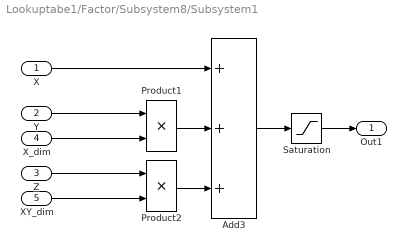
== system Lookuptabe1/Factor/Subsystem8/Subsystem1 ==
  X : Inport
  Y : Inport  Port=2
  Z : Inport  Port=3
  X_dim : Inport  Port=4
  XY_dim : Inport  Port=5
  Add3 : Sum  Inputs=3  OutDataTypeStr=uint16
  Product1 : Product  OutDataTypeStr=uint16
  Product2 : Product  OutDataTypeStr=uint16
  Saturation : Saturate  UpperLimit=X_dim*Y_dim*Z_dim-1  LowerLimit=0
  Out1 : Outport  VectorParamsAs1DForOutWhenUnconnected=off
  wires:
  Product1/1 -> Add3/2
  Add3/1 -> Saturation/1
  X_dim/1 -> Product1/2
  X/1 -> Add3/1
  Y/1 -> Product1/1
  Saturation/1 -> Out1/1
  XY_dim/1 -> Product2/2
  Z/1 -> Product2/1
  Product2/1 -> Add3/3

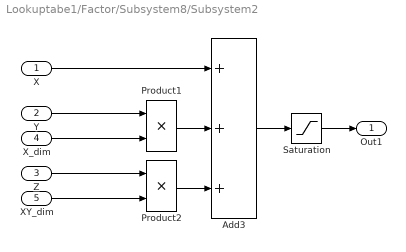
== system Lookuptabe1/Factor/Subsystem8/Subsystem2 ==
  X : Inport
  Y : Inport  Port=2
  Z : Inport  Port=3
  X_dim : Inport  Port=4
  XY_dim : Inport  Port=5
  Add3 : Sum  Inputs=3  OutDataTypeStr=uint16
  Product1 : Product  OutDataTypeStr=uint16
  Product2 : Product  OutDataTypeStr=uint16
  Saturation : Saturate  UpperLimit=X_dim*Y_dim*Z_dim-1  LowerLimit=0
  Out1 : Outport  VectorParamsAs1DForOutWhenUnconnected=off
  wires:
  Product2/1 -> Add3/3
  Z/1 -> Product2/1
  XY_dim/1 -> Product2/2
  Saturation/1 -> Out1/1
  Y/1 -> Product1/1
  X/1 -> Add3/1
  X_dim/1 -> Product1/2
  Add3/1 -> Saturation/1
  Product1/1 -> Add3/2

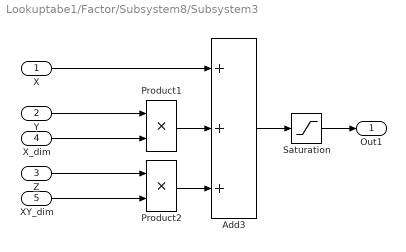
== system Lookuptabe1/Factor/Subsystem8/Subsystem3 ==
  X : Inport
  Y : Inport  Port=2
  Z : Inport  Port=3
  X_dim : Inport  Port=4
  XY_dim : Inport  Port=5
  Add3 : Sum  Inputs=3  OutDataTypeStr=uint16
  Product1 : Product  OutDataTypeStr=uint16
  Product2 : Product  OutDataTypeStr=uint16
  Saturation : Saturate  UpperLimit=X_dim*Y_dim*Z_dim-1  LowerLimit=0
  Out1 : Outport  VectorParamsAs1DForOutWhenUnconnected=off
  wires:
  Product1/1 -> Add3/2
  Add3/1 -> Saturation/1
  X_dim/1 -> Product1/2
  X/1 -> Add3/1
  Y/1 -> Product1/1
  Saturation/1 -> Out1/1
  XY_dim/1 -> Product2/2
  Z/1 -> Product2/1
  Product2/1 -> Add3/3

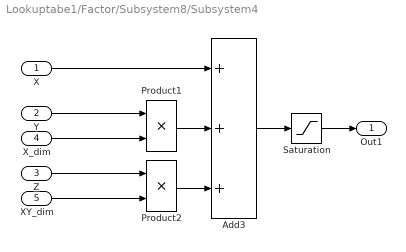
== system Lookuptabe1/Factor/Subsystem8/Subsystem4 ==
  X : Inport
  Y : Inport  Port=2
  Z : Inport  Port=3
  X_dim : Inport  Port=4
  XY_dim : Inport  Port=5
  Add3 : Sum  Inputs=3  OutDataTypeStr=uint16
  Product1 : Product  OutDataTypeStr=uint16
  Product2 : Product  OutDataTypeStr=uint16
  Saturation : Saturate  UpperLimit=X_dim*Y_dim*Z_dim-1  LowerLimit=0
  Out1 : Outport  VectorParamsAs1DForOutWhenUnconnected=off
  wires:
  Product2/1 -> Add3/3
  Z/1 -> Product2/1
  XY_dim/1 -> Product2/2
  Saturation/1 -> Out1/1
  Y/1 -> Product1/1
  X/1 -> Add3/1
  X_dim/1 -> Product1/2
  Add3/1 -> Saturation/1
  Product1/1 -> Add3/2

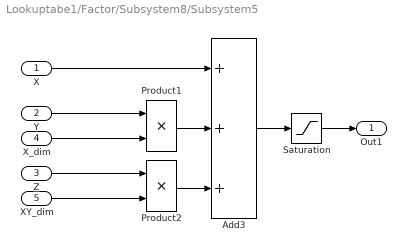
== system Lookuptabe1/Factor/Subsystem8/Subsystem5 ==
  X : Inport
  Y : Inport  Port=2
  Z : Inport  Port=3
  X_dim : Inport  Port=4
  XY_dim : Inport  Port=5
  Add3 : Sum  Inputs=3  OutDataTypeStr=uint16
  Product1 : Product  OutDataTypeStr=uint16
  Product2 : Product  OutDataTypeStr=uint16
  Saturation : Saturate  UpperLimit=X_dim*Y_dim*Z_dim-1  LowerLimit=0
  Out1 : Outport  VectorParamsAs1DForOutWhenUnconnected=off
  wires:
  Product1/1 -> Add3/2
  Add3/1 -> Saturation/1
  X_dim/1 -> Product1/2
  X/1 -> Add3/1
  Y/1 -> Product1/1
  Saturation/1 -> Out1/1
  XY_dim/1 -> Product2/2
  Z/1 -> Product2/1
  Product2/1 -> Add3/3

== system Lookuptabe1/Factor/Subsystem8/Subsystem6 ==
  X : Inport
  Y : Inport  Port=2
  Z : Inport  Port=3
  X_dim : Inport  Port=4
  XY_dim : Inport  Port=5
  Add3 : Sum  Inputs=3  OutDataTypeStr=uint16
  Product1 : Product  OutDataTypeStr=uint16
  Product2 : Product  OutDataTypeStr=uint16
  Saturation : Saturate  UpperLimit=X_dim*Y_dim*Z_dim-1  LowerLimit=0
  Out1 : Outport  VectorParamsAs1DForOutWhenUnconnected=off
  wires:
  Product2/1 -> Add3/3
  Z/1 -> Product2/1
  XY_dim/1 -> Product2/2
  Saturation/1 -> Out1/1
  Y/1 -> Product1/1
  X/1 -> Add3/1
  X_dim/1 -> Product1/2
  Add3/1 -> Saturation/1
  Product1/1 -> Add3/2

== system Lookuptabe1/Factor/Subsystem8/Subsystem7 ==
  X : Inport
  Y : Inport  Port=2
  Z : Inport  Port=3
  X_dim : Inport  Port=4
  XY_dim : Inport  Port=5
  Add3 : Sum  Inputs=3  OutDataTypeStr=uint16
  Product1 : Product  OutDataTypeStr=uint16
  Product2 : Product  OutDataTypeStr=uint16
  Saturation : Saturate  UpperLimit=X_dim*Y_dim*Z_dim-1  LowerLimit=0
  Out1 : Outport  VectorParamsAs1DForOutWhenUnconnected=off
  wires:
  Product1/1 -> Add3/2
  Add3/1 -> Saturation/1
  X_dim/1 -> Product1/2
  X/1 -> Add3/1
  Y/1 -> Product1/1
  Saturation/1 -> Out1/1
  XY_dim/1 -> Product2/2
  Z/1 -> Product2/1
  Product2/1 -> Add3/3

== system Lookuptabe1/Factor/Subsystem8/Subsystem8 ==
  X : Inport
  Y : Inport  Port=2
  Z : Inport  Port=3
  X_dim : Inport  Port=4
  XY_dim : Inport  Port=5
  Add3 : Sum  Inputs=3  OutDataTypeStr=uint16
  Product1 : Product  OutDataTypeStr=uint16
  Product2 : Product  OutDataTypeStr=uint16
  Saturation : Saturate  UpperLimit=X_dim*Y_dim*Z_dim-1  LowerLimit=0
  Out1 : Outport  VectorParamsAs1DForOutWhenUnconnected=off
  wires:
  Product2/1 -> Add3/3
  Z/1 -> Product2/1
  XY_dim/1 -> Product2/2
  Saturation/1 -> Out1/1
  Y/1 -> Product1/1
  X/1 -> Add3/1
  X_dim/1 -> Product1/2
  Add3/1 -> Saturation/1
  Product1/1 -> Add3/2

== system Lookuptabe1/Factor/Factor/Subsystem8/Subsystem1 ==
  X : Inport
  Y : Inport  Port=2
  Z : Inport  Port=3
  X_dim : Inport  Port=4
  XY_dim : Inport  Port=5
  Add3 : Sum  Inputs=3  OutDataTypeStr=uint16
  Product1 : Product  OutDataTypeStr=double
  Product2 : Product
  Saturation : Saturate  UpperLimit=X_dim*Y_dim*Z_dim-1  LowerLimit=0  OutDataTypeStr=single
  Out1 : Outport  VectorParamsAs1DForOutWhenUnconnected=off
  wires:
  Product2/1 -> Add3/3
  Z/1 -> Product2/1
  XY_dim/1 -> Product2/2
  Saturation/1 -> Out1/1
  Y/1 -> Product1/1
  X/1 -> Add3/1
  X_dim/1 -> Product1/2
  Add3/1 -> Saturation/1
  Product1/1 -> Add3/2

== system Lookuptabe1/Factor/Factor/Subsystem8/Subsystem2 ==
  X : Inport
  Y : Inport  Port=2
  Z : Inport  Port=3
  X_dim : Inport  Port=4
  XY_dim : Inport  Port=5
  Add3 : Sum  Inputs=3  OutDataTypeStr=uint16
  Product1 : Product  OutDataTypeStr=double
  Product2 : Product
  Saturation : Saturate  UpperLimit=X_dim*Y_dim*Z_dim-1  LowerLimit=0  OutDataTypeStr=single
  Out1 : Outport  VectorParamsAs1DForOutWhenUnconnected=off
  wires:
  Product2/1 -> Add3/3
  Z/1 -> Product2/1
  XY_dim/1 -> Product2/2
  Saturation/1 -> Out1/1
  Y/1 -> Product1/1
  X/1 -> Add3/1
  X_dim/1 -> Product1/2
  Add3/1 -> Saturation/1
  Product1/1 -> Add3/2

== system Lookuptabe1/Factor/Factor/Subsystem8/Subsystem3 ==
  X : Inport
  Y : Inport  Port=2
  Z : Inport  Port=3
  X_dim : Inport  Port=4
  XY_dim : Inport  Port=5
  Add3 : Sum  Inputs=3  OutDataTypeStr=uint16
  Product1 : Product  OutDataTypeStr=double
  Product2 : Product
  Saturation : Saturate  UpperLimit=X_dim*Y_dim*Z_dim-1  LowerLimit=0  OutDataTypeStr=single
  Out1 : Outport  VectorParamsAs1DForOutWhenUnconnected=off
  wires:
  Product2/1 -> Add3/3
  Z/1 -> Product2/1
  XY_dim/1 -> Product2/2
  Saturation/1 -> Out1/1
  Y/1 -> Product1/1
  X/1 -> Add3/1
  X_dim/1 -> Product1/2
  Add3/1 -> Saturation/1
  Product1/1 -> Add3/2

== system Lookuptabe1/Factor/Factor/Subsystem8/Subsystem4 ==
  X : Inport
  Y : Inport  Port=2
  Z : Inport  Port=3
  X_dim : Inport  Port=4
  XY_dim : Inport  Port=5
  Add3 : Sum  Inputs=3  OutDataTypeStr=uint16
  Product1 : Product  OutDataTypeStr=double
  Product2 : Product
  Saturation : Saturate  UpperLimit=X_dim*Y_dim*Z_dim-1  LowerLimit=0  OutDataTypeStr=single
  Out1 : Outport  VectorParamsAs1DForOutWhenUnconnected=off
  wires:
  Product2/1 -> Add3/3
  Z/1 -> Product2/1
  XY_dim/1 -> Product2/2
  Saturation/1 -> Out1/1
  Y/1 -> Product1/1
  X/1 -> Add3/1
  X_dim/1 -> Product1/2
  Add3/1 -> Saturation/1
  Product1/1 -> Add3/2

== system Lookuptabe1/Factor/Factor/Subsystem8/Subsystem5 ==
  X : Inport
  Y : Inport  Port=2
  Z : Inport  Port=3
  X_dim : Inport  Port=4
  XY_dim : Inport  Port=5
  Add3 : Sum  Inputs=3  OutDataTypeStr=uint16
  Product1 : Product  OutDataTypeStr=double
  Product2 : Product
  Saturation : Saturate  UpperLimit=X_dim*Y_dim*Z_dim-1  LowerLimit=0  OutDataTypeStr=single
  Out1 : Outport  VectorParamsAs1DForOutWhenUnconnected=off
  wires:
  Product2/1 -> Add3/3
  Z/1 -> Product2/1
  XY_dim/1 -> Product2/2
  Saturation/1 -> Out1/1
  Y/1 -> Product1/1
  X/1 -> Add3/1
  X_dim/1 -> Product1/2
  Add3/1 -> Saturation/1
  Product1/1 -> Add3/2

== system Lookuptabe1/Factor/Factor/Subsystem8/Subsystem6 ==
  X : Inport
  Y : Inport  Port=2
  Z : Inport  Port=3
  X_dim : Inport  Port=4
  XY_dim : Inport  Port=5
  Add3 : Sum  Inputs=3  OutDataTypeStr=uint16
  Product1 : Product  OutDataTypeStr=double
  Product2 : Product
  Saturation : Saturate  UpperLimit=X_dim*Y_dim*Z_dim-1  LowerLimit=0  OutDataTypeStr=single
  Out1 : Outport  VectorParamsAs1DForOutWhenUnconnected=off
  wires:
  Product2/1 -> Add3/3
  Z/1 -> Product2/1
  XY_dim/1 -> Product2/2
  Saturation/1 -> Out1/1
  Y/1 -> Product1/1
  X/1 -> Add3/1
  X_dim/1 -> Product1/2
  Add3/1 -> Saturation/1
  Product1/1 -> Add3/2

== system Lookuptabe1/Factor/Factor/Subsystem8/Subsystem7 ==
  X : Inport
  Y : Inport  Port=2
  Z : Inport  Port=3
  X_dim : Inport  Port=4
  XY_dim : Inport  Port=5
  Add3 : Sum  Inputs=3  OutDataTypeStr=uint16
  Product1 : Product  OutDataTypeStr=double
  Product2 : Product
  Saturation : Saturate  UpperLimit=X_dim*Y_dim*Z_dim-1  LowerLimit=0  OutDataTypeStr=single
  Out1 : Outport  VectorParamsAs1DForOutWhenUnconnected=off
  wires:
  Product2/1 -> Add3/3
  Z/1 -> Product2/1
  XY_dim/1 -> Product2/2
  Saturation/1 -> Out1/1
  Y/1 -> Product1/1
  X/1 -> Add3/1
  X_dim/1 -> Product1/2
  Add3/1 -> Saturation/1
  Product1/1 -> Add3/2

== system Lookuptabe1/Factor/Factor/Subsystem8/Subsystem8 ==
  X : Inport
  Y : Inport  Port=2
  Z : Inport  Port=3
  X_dim : Inport  Port=4
  XY_dim : Inport  Port=5
  Add3 : Sum  Inputs=3  OutDataTypeStr=uint16
  Product1 : Product  OutDataTypeStr=uint16
  Product2 : Product  OutDataTypeStr=uint16
  Saturation : Saturate  UpperLimit=X_dim*Y_dim*Z_dim-1  LowerLimit=0  OutDataTypeStr=single
  Out1 : Outport  VectorParamsAs1DForOutWhenUnconnected=off
  wires:
  Product1/1 -> Add3/2
  Add3/1 -> Saturation/1
  X_dim/1 -> Product1/2
  X/1 -> Add3/1
  Y/1 -> Product1/1
  Saturation/1 -> Out1/1
  XY_dim/1 -> Product2/2
  Z/1 -> Product2/1
  Product2/1 -> Add3/3

== system Lookuptabe1/Factor/Id Lookup Table1/Subsystem8/Subsystem1 ==
  X : Inport
  Y : Inport  Port=2
  Z : Inport  Port=3
  X_dim : Inport  Port=4
  XY_dim : Inport  Port=5
  Add3 : Sum  Inputs=3  OutDataTypeStr=uint16
  Product1 : Product  OutDataTypeStr=double
  Product2 : Product
  Saturation : Saturate  UpperLimit=X_dim*Y_dim*Z_dim-1  LowerLimit=0  OutDataTypeStr=single
  Out1 : Outport  VectorParamsAs1DForOutWhenUnconnected=off
  wires:
  Product1/1 -> Add3/2
  Add3/1 -> Saturation/1
  X_dim/1 -> Product1/2
  X/1 -> Add3/1
  Y/1 -> Product1/1
  Saturation/1 -> Out1/1
  XY_dim/1 -> Product2/2
  Z/1 -> Product2/1
  Product2/1 -> Add3/3

== system Lookuptabe1/Factor/Id Lookup Table1/Subsystem8/Subsystem2 ==
  X : Inport
  Y : Inport  Port=2
  Z : Inport  Port=3
  X_dim : Inport  Port=4
  XY_dim : Inport  Port=5
  Add3 : Sum  Inputs=3  OutDataTypeStr=uint16
  Product1 : Product  OutDataTypeStr=double
  Product2 : Product
  Saturation : Saturate  UpperLimit=X_dim*Y_dim*Z_dim-1  LowerLimit=0  OutDataTypeStr=single
  Out1 : Outport  VectorParamsAs1DForOutWhenUnconnected=off
  wires:
  Product1/1 -> Add3/2
  Add3/1 -> Saturation/1
  X_dim/1 -> Product1/2
  X/1 -> Add3/1
  Y/1 -> Product1/1
  Saturation/1 -> Out1/1
  XY_dim/1 -> Product2/2
  Z/1 -> Product2/1
  Product2/1 -> Add3/3

== system Lookuptabe1/Factor/Id Lookup Table1/Subsystem8/Subsystem3 ==
  X : Inport
  Y : Inport  Port=2
  Z : Inport  Port=3
  X_dim : Inport  Port=4
  XY_dim : Inport  Port=5
  Add3 : Sum  Inputs=3  OutDataTypeStr=uint16
  Product1 : Product  OutDataTypeStr=double
  Product2 : Product
  Saturation : Saturate  UpperLimit=X_dim*Y_dim*Z_dim-1  LowerLimit=0  OutDataTypeStr=single
  Out1 : Outport  VectorParamsAs1DForOutWhenUnconnected=off
  wires:
  Product1/1 -> Add3/2
  Add3/1 -> Saturation/1
  X_dim/1 -> Product1/2
  X/1 -> Add3/1
  Y/1 -> Product1/1
  Saturation/1 -> Out1/1
  XY_dim/1 -> Product2/2
  Z/1 -> Product2/1
  Product2/1 -> Add3/3

== system Lookuptabe1/Factor/Id Lookup Table1/Subsystem8/Subsystem4 ==
  X : Inport
  Y : Inport  Port=2
  Z : Inport  Port=3
  X_dim : Inport  Port=4
  XY_dim : Inport  Port=5
  Add3 : Sum  Inputs=3  OutDataTypeStr=uint16
  Product1 : Product  OutDataTypeStr=double
  Product2 : Product
  Saturation : Saturate  UpperLimit=X_dim*Y_dim*Z_dim-1  LowerLimit=0  OutDataTypeStr=single
  Out1 : Outport  VectorParamsAs1DForOutWhenUnconnected=off
  wires:
  Product1/1 -> Add3/2
  Add3/1 -> Saturation/1
  X_dim/1 -> Product1/2
  X/1 -> Add3/1
  Y/1 -> Product1/1
  Saturation/1 -> Out1/1
  XY_dim/1 -> Product2/2
  Z/1 -> Product2/1
  Product2/1 -> Add3/3

== system Lookuptabe1/Factor/Id Lookup Table1/Subsystem8/Subsystem5 ==
  X : Inport
  Y : Inport  Port=2
  Z : Inport  Port=3
  X_dim : Inport  Port=4
  XY_dim : Inport  Port=5
  Add3 : Sum  Inputs=3  OutDataTypeStr=uint16
  Product1 : Product  OutDataTypeStr=double
  Product2 : Product
  Saturation : Saturate  UpperLimit=X_dim*Y_dim*Z_dim-1  LowerLimit=0  OutDataTypeStr=single
  Out1 : Outport  VectorParamsAs1DForOutWhenUnconnected=off
  wires:
  Product1/1 -> Add3/2
  Add3/1 -> Saturation/1
  X_dim/1 -> Product1/2
  X/1 -> Add3/1
  Y/1 -> Product1/1
  Saturation/1 -> Out1/1
  XY_dim/1 -> Product2/2
  Z/1 -> Product2/1
  Product2/1 -> Add3/3

== system Lookuptabe1/Factor/Id Lookup Table1/Subsystem8/Subsystem6 ==
  X : Inport
  Y : Inport  Port=2
  Z : Inport  Port=3
  X_dim : Inport  Port=4
  XY_dim : Inport  Port=5
  Add3 : Sum  Inputs=3  OutDataTypeStr=uint16
  Product1 : Product  OutDataTypeStr=double
  Product2 : Product
  Saturation : Saturate  UpperLimit=X_dim*Y_dim*Z_dim-1  LowerLimit=0  OutDataTypeStr=single
  Out1 : Outport  VectorParamsAs1DForOutWhenUnconnected=off
  wires:
  Product1/1 -> Add3/2
  Add3/1 -> Saturation/1
  X_dim/1 -> Product1/2
  X/1 -> Add3/1
  Y/1 -> Product1/1
  Saturation/1 -> Out1/1
  XY_dim/1 -> Product2/2
  Z/1 -> Product2/1
  Product2/1 -> Add3/3

== system Lookuptabe1/Factor/Id Lookup Table1/Subsystem8/Subsystem7 ==
  X : Inport
  Y : Inport  Port=2
  Z : Inport  Port=3
  X_dim : Inport  Port=4
  XY_dim : Inport  Port=5
  Add3 : Sum  Inputs=3  OutDataTypeStr=uint16
  Product1 : Product  OutDataTypeStr=double
  Product2 : Product
  Saturation : Saturate  UpperLimit=X_dim*Y_dim*Z_dim-1  LowerLimit=0  OutDataTypeStr=single
  Out1 : Outport  VectorParamsAs1DForOutWhenUnconnected=off
  wires:
  Product1/1 -> Add3/2
  Add3/1 -> Saturation/1
  X_dim/1 -> Product1/2
  X/1 -> Add3/1
  Y/1 -> Product1/1
  Saturation/1 -> Out1/1
  XY_dim/1 -> Product2/2
  Z/1 -> Product2/1
  Product2/1 -> Add3/3

== system Lookuptabe1/Factor/Id Lookup Table1/Subsystem8/Subsystem8 ==
  X : Inport
  Y : Inport  Port=2
  Z : Inport  Port=3
  X_dim : Inport  Port=4
  XY_dim : Inport  Port=5
  Add3 : Sum  Inputs=3  OutDataTypeStr=uint16
  Product1 : Product  OutDataTypeStr=uint16
  Product2 : Product  OutDataTypeStr=uint16
  Saturation : Saturate  UpperLimit=X_dim*Y_dim*Z_dim-1  LowerLimit=0  OutDataTypeStr=single
  Out1 : Outport  VectorParamsAs1DForOutWhenUnconnected=off
  wires:
  Product2/1 -> Add3/3
  Z/1 -> Product2/1
  XY_dim/1 -> Product2/2
  Saturation/1 -> Out1/1
  Y/1 -> Product1/1
  X/1 -> Add3/1
  X_dim/1 -> Product1/2
  Add3/1 -> Saturation/1
  Product1/1 -> Add3/2
